simulink model "SERVOMOTOR_RESONANTLOAD"  (R2024b)
settings: Solver=VariableStepAuto  StartTime=0.0  StopTime=10.0  RelTol=1e-3
values from neighbouring files (symbols this model uses):
  denDriv = [Tdrv 1]    [simulation.m]
  numDriv = [kdrv]    [simulation.m]
undefined symbols (not defined in the file or in its folder): daq, drv, sens
settings Model: Creator=llp  LastModifiedBy=llp

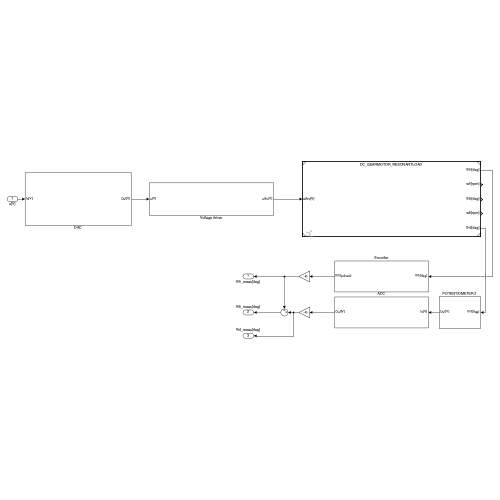
[thumbnail: Simulink's stored preview of the top-level diagram]
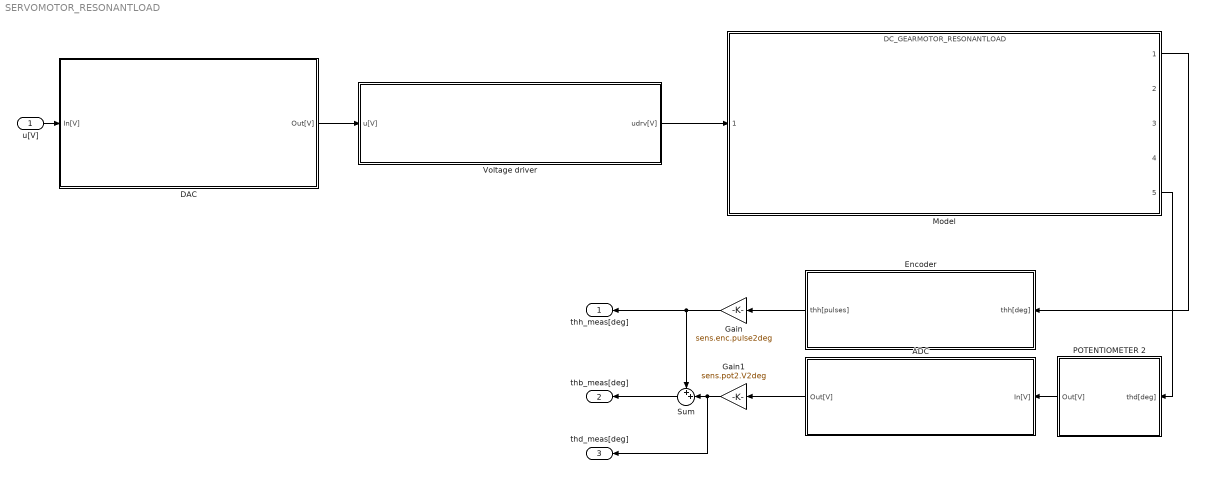
== system SERVOMOTOR_RESONANTLOAD ==
  u[V] : Inport
  ADC : Subsystem
  DAC : Subsystem
  Encoder : Subsystem
  Gain : Gain  Gain=sens.enc.pulse2deg
  Gain1 : Gain  Gain=sens.pot2.V2deg
  Model : ModelReference  ModelNameDialog=DC_GEARMOTOR_RESONANTLOAD.slx  SimulationMode=Normal  ModelReferenceVersion=1.6
  POTENTIOMETER 2 : Subsystem
  Sum : Sum  Inputs=++|
  Voltage driver : Subsystem
  thh_meas[deg] : Outport
  thb_meas[deg] : Outport  Port=2
  thd_meas[deg] : Outport  Port=3
  wires:
  u[V]/1 -> DAC/1(In[V])
  Encoder/1(thh[pulses]) -> Gain/1
  DAC/1(Out[V]) -> Voltage driver/1(u[V])
  Voltage driver/1(udrv[V]) -> Model/1
  Gain/1 -> Sum/1, thh_meas[deg]/1
  Sum/1 -> thb_meas[deg]/1
  Gain1/1 -> thd_meas[deg]/1, Sum/2
  Model/1 -> Encoder/1(thh[deg])
  Model/5 -> POTENTIOMETER 2/1(thd[deg])
  POTENTIOMETER 2/1(Out[V]) -> ADC/1(In[V])
  ADC/1(Out[V]) -> Gain1/1

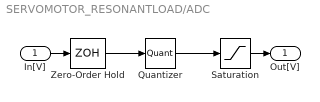
== system SERVOMOTOR_RESONANTLOAD/ADC ==
  In[V] : Inport
  Quantizer : Quantizer  QuantizationInterval=daq.adc.q
  Saturation : Saturate  UpperLimit=daq.adc.fs  LowerLimit=-daq.adc.fs
  Zero-Order Hold : ZeroOrderHold  SampleTime=daq.adc.ts
  Out[V] : Outport
  wires:
  Saturation/1 -> Out[V]/1
  In[V]/1 -> Zero-Order Hold/1
  Zero-Order Hold/1 -> Quantizer/1
  Quantizer/1 -> Saturation/1

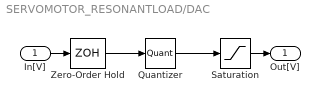
== system SERVOMOTOR_RESONANTLOAD/DAC ==
  In[V] : Inport
  Quantizer : Quantizer  QuantizationInterval=daq.dac.q
  Saturation : Saturate  UpperLimit=daq.dac.fs  LowerLimit=-daq.dac.fs
  Zero-Order Hold : ZeroOrderHold  SampleTime=daq.dac.ts
  Out[V] : Outport
  wires:
  Saturation/1 -> Out[V]/1
  In[V]/1 -> Zero-Order Hold/1
  Zero-Order Hold/1 -> Quantizer/1
  Quantizer/1 -> Saturation/1

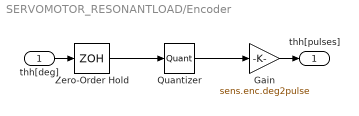
== system SERVOMOTOR_RESONANTLOAD/Encoder ==
  thh[deg] : Inport
  Gain : Gain  Gain=sens.enc.deg2pulse
  Quantizer : Quantizer  QuantizationInterval=daq.adc.q
  Zero-Order Hold : ZeroOrderHold  SampleTime=daq.adc.ts
  thh[pulses] : Outport
  wires:
  thh[deg]/1 -> Zero-Order Hold/1
  Gain/1 -> thh[pulses]/1
  Quantizer/1 -> Gain/1
  Zero-Order Hold/1 -> Quantizer/1

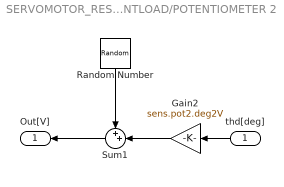
== system SERVOMOTOR_RESONANTLOAD/POTENTIOMETER 2 ==
  thd[deg] : Inport
  Gain2 : Gain  Gain=sens.pot2.deg2V
  Random Number : RandomNumber  Variance=sens.pot2.noise.var  SampleTime=sens.pot2.Ts
  Sum1 : Sum  Inputs=++|
  Out[V] : Outport
  wires:
  thd[deg]/1 -> Gain2/1
  Gain2/1 -> Sum1/2
  Random Number/1 -> Sum1/1
  Sum1/1 -> Out[V]/1

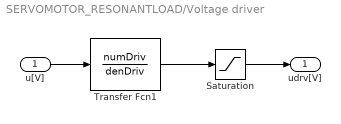
== system SERVOMOTOR_RESONANTLOAD/Voltage driver ==
  u[V] : Inport
  Saturation : Saturate  UpperLimit=drv.outmax  LowerLimit=-drv.outmax
  Transfer Fcn1 : TransferFcn  Numerator=numDriv  Denominator=denDriv
  udrv[V] : Outport
  wires:
  u[V]/1 -> Transfer Fcn1/1
  Saturation/1 -> udrv[V]/1
  Transfer Fcn1/1 -> Saturation/1
